simulink model "MotorGenerator1Basic_test_harness"  (R2022a)
settings: Solver=ode23t  StartTime=0.0  StopTime=t_end  RelTol=1e-3  AbsTol=1e-3
PreLoadFcn:
  | MotorGenerator1Basic_setup
undefined symbols (not defined in the file or in its folder): testharness
libraries: nesl_utility x3, fl_lib x1, sdl_lib x1
settings Model: Creator=isaacito  LastModifiedBy=isaacito
settings SolverCC: AutoScaleAbsTol=off  AlgebraicLoopSolver=TrustRegion
settings DebuggingCC: UnconnectedInputMsg=warning  UnconnectedOutputMsg=warning  UnconnectedLineMsg=warning  SymbolicDimsDataTypeCodeGenerationDiagnostic=none  SFMachineParentedDataDiag=warning
settings SFSimCC: CustomCodeUndefinedFunction=UseInterfaceOnly
settings RTWCC: DLArmComputeVersion=19.05
settings SimscapeCC: SimscapeLogType=all  SimscapeLogSimulationStatistics=on  SimscapeLogLimitData=off  SimscapeLogDataHistory=10000

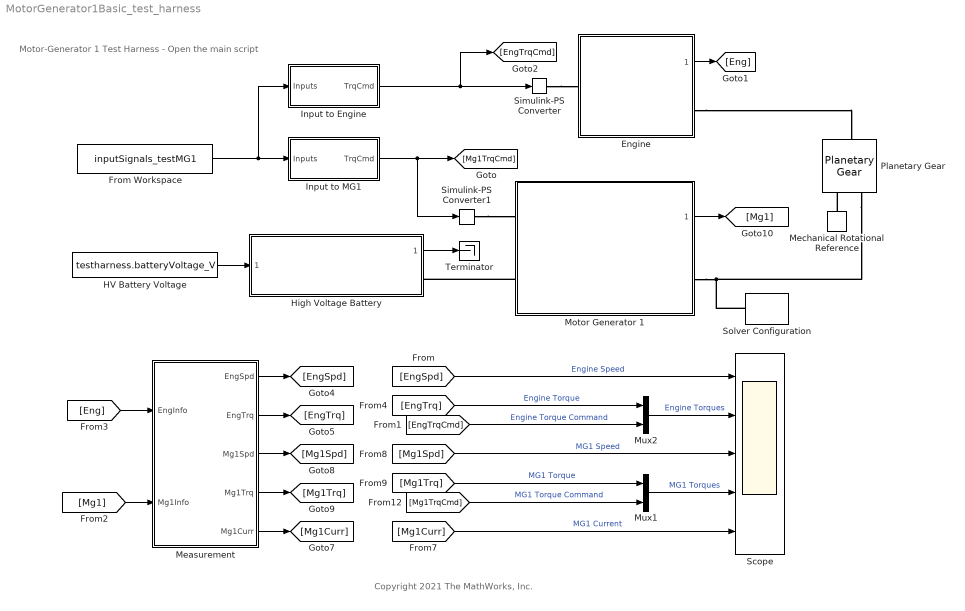
== system MotorGenerator1Basic_test_harness ==
  note: Copyright 2021 The MathWorks, Inc.
  note: Motor-Generator 1 Test Harness
      | - Open the main script
  Engine : Subsystem  ReferencedSubsystem=EngineBasic_refsub
      settings: PortSchema="{\"entries\":[{\"content\":{\"sides\":[{\"content\":{\"connectorIds\":[\"RConn1\"]},\"type\":\"ConnectorPlacement.EquallySpacedRectSide\",\"uuid\":\"5f0e7c9a-363d-4994-a013-d94ca7bd087a\"},{\"content\":{\"connectorIds\":[\"Out1\",\"LConn1\"],\"side\":\"RIGHT\"},\"type\":\"ConnectorPlacement.EquallySpacedRectSide\",\"uuid\":\"ebc3b24e-2640-42e1-8db7-715085fcccfd\"},{\"content\":{\"connectorIds\":[],\"side\":\"TOP\"},\"type\":\"ConnectorPlacement.EquallySpacedRectSide\",\"uuid\":\"348bf4c7-11ba-4351-a8af-87d33bf26f7f\"},{\"content\":{\"connectorIds\":[],\"side\":\"HIDDEN\"},\"type\":\"ConnectorPlacement.EquallySpacedRectSide\",\"uuid\":\"1cb82837-ca80-45c4-bec7-ac28580eadb7\"}]},\"type\":\"ConnectorPlacement.EquallySpacedConnector\",\"uuid\":\"6e937982-b0a5-454c-84b0-bd79245ef5fe\"}],\"packageUris\":[\"http://schema.mathworks.com/mf0/Connector/R2020b\"],\"version\":\"1.0\"}"
  From Workspace : FromWorkspace  VariableName=inputSignals_testMG1  OutDataTypeStr=Bus: inputBus_testMG1  Interpolate=off  OutputAfterFinalValue=Holding final value
      settings: AttributesFormatString=%<OutDataTypeStr>
  HV Battery Voltage : Constant  Value=testharness.batteryVoltage_V
  High Voltage Battery : Subsystem  ReferencedSubsystem=BatteryForTest_refsub
  Input to Engine : Subsystem
  Input to MG1 : Subsystem
  Measurement : Subsystem
  Mechanical Rotational Reference : fl_lib/Mechanical/Rotational Elements/Mechanical Rotational Reference
      settings: SourceProductBaseCode=PW,SS,VE
  Motor Generator 1 : Subsystem  ReferencedSubsystem=MotorGenerator1Basic_refsub
      settings: PortSchema="{\"entries\":[{\"content\":{\"sides\":[{\"content\":{\"connectorIds\":[\"LConn2\",\"LConn1\"]},\"type\":\"ConnectorPlacement.EquallySpacedRectSide\",\"uuid\":\"776eba5b-fa0b-476e-bc25-638ffdaad34f\"},{\"content\":{\"connectorIds\":[\"Out1\",\"RConn1\"],\"side\":\"RIGHT\"},\"type\":\"ConnectorPlacement.EquallySpacedRectSide\",\"uuid\":\"4f3a20f1-a757-4d58-af45-1ca561c570ae\"},{\"content\":{\"connectorIds\":[],\"side\":\"TOP\"},\"type\":\"ConnectorPlacement.EquallySpacedRectSide\",\"uuid\":\"92ea57c0-7c62-4e58-98f6-e0ae25305e81\"},{\"content\":{\"connectorIds\":[],\"side\":\"HIDDEN\"},\"type\":\"ConnectorPlacement.EquallySpacedRectSide\",\"uuid\":\"c19be4f7-c21d-4f93-a091-e01cfe3eb863\"}]},\"type\":\"ConnectorPlacement.EquallySpacedConnector\",\"uuid\":\"27ec3241-2d74-4878-8a97-99674a624e01\"}],\"packageUris\":[\"http://schema.mathworks.com/mf0/Connector/R2020b\"],\"version\":\"1.0\"}"
  Mux1 : Mux  Inputs=2
  Mux2 : Mux  Inputs=2
  Planetary Gear : sdl_lib/Gears/Planetary Gear  rs_ratio=powerSplit.planetary_ringToSunGearRatio  friction_model=sdl.enum.gear_friction.constant  efficiency=powerSplit.planetary_efficiencies  temperature_TLU=[280, 300, 320] K  efficiency_sp_TLU=[.95, .9, .85]  efficiency_rp_TLU=[.95, .9, .85]  pwr_thr=smoothing.planetary_meshing_loss_thresholds_W W  mu_visc=powerSplit.planetary_frictions_Nm_per_rpm m*N/rpm  model_inertia=simscape.enum.onoff.on  planet_inertia=powerSplit.planetary_planetGearInertia_kg_m2 kg*m^2  thermal_mass=50 J/K  T_init=300 K
      settings: SourceProductBaseCode=LD
  Scope : Scope  NumInputPorts=5
  Simulink-PS Converter : nesl_utility/Simulink-PS Converter  PhysicalDomain=network_engine_domain  SubClassName=ps_input  LeftPortType=input  RightPortType=output  PseudoPeriodic=off  Frequencies=[]  NoiseDistribution=none  NoiseParameters=[]  Unit=N*m  AffineConversion=off  FilteringAndDerivatives=provide  SimscapeFilterOrder=1  InputFilterTimeConstant=0.001  UdotUserProvided=0
      settings: SourceProductName=Utilities
  Simulink-PS Converter1 : nesl_utility/Simulink-PS Converter  PhysicalDomain=network_engine_domain  SubClassName=ps_input  LeftPortType=input  RightPortType=output  PseudoPeriodic=off  Frequencies=[]  NoiseDistribution=none  NoiseParameters=[]  Unit=N*m  AffineConversion=off  FilteringAndDerivatives=provide  SimscapeFilterOrder=1  InputFilterTimeConstant=0.001  UdotUserProvided=0
      settings: SourceProductName=Utilities
  Solver Configuration : nesl_utility/Solver Configuration  PhysicalDomain=network_engine_domain  SubClassName=solver  LeftPortType=input  RightPortType=generic  Tones=[]  Harmonics=[]  SimulateNoise=off  Profile=off  UseLocalSampling=off  EnableSwitchedLinearOptims=on  FrequencyDomain=off  UseCCode=off  RelTol=0.001  AbsTol=1e-06  MinStep=1e-09  ToWorkspace=off  RevertToSquareIcSolve=off  NumHomotopyIterations=100  PhasorMode=off  PhasorModeNumHarmonics=1  IndexReductionMethod=DerivativeReplacement  DoDC=off  ResidualTolerance=1e-09  UseLocalSolver=off  LocalSolverChoice=NE_BACKWARD_EULER_ADVANCER  LocalSolverSampleTime=0.001  DoFixedCost=off  MaxNonlinIter=3  MaxModeIter=2  ComputeImpulses=off  ImpulseIterations=2  LinearAlgebra=auto  LinearAlgebraNumThread=0  EquationFormulation=NE_TIME_EF  DelaysMemoryBudget=1024  AutomaticFiltering=on  FilteringTimeConstant=0.001  PartitionStorageMethod=AS_NEEDED  PartitionMemoryBudget=1024  PartitionMethod=ROBUST
      settings: SourceProductName=Utilities
  Terminator : Terminator
  wires:
  HV Battery Voltage/1 -> High Voltage Battery/1
  [Eng] -> Measurement/1(EngInfo)
  [Mg1] -> Measurement/2(Mg1Info)
  Measurement/1(EngSpd) -> [EngSpd]
  Measurement/2(EngTrq) -> [EngTrq]
  Measurement/5(Mg1Curr) -> [Mg1Curr]
  Measurement/3(Mg1Spd) -> [Mg1Spd]
  Measurement/4(Mg1Trq) -> [Mg1Trq]
  [Mg1TrqCmd] -> Mux1/2  "MG1 Torque Command"
  [Mg1Trq] -> Mux1/1  "MG1 Torque"
  Input to Engine/1(TrqCmd) -> [EngTrqCmd], Simulink-PS Converter/1
  Engine/1 -> [Eng]
  [EngTrq] -> Mux2/1  "Engine Torque"
  [EngTrqCmd] -> Mux2/2  "Engine Torque Command"
  [EngSpd] -> Scope/1  "Engine Speed"
  Mux2/1 -> Scope/2  "Engine Torques"
  Mux1/1 -> Scope/4  "MG1 Torques"
  [Mg1Curr] -> Scope/5  "MG1 Current"
  From Workspace/1 -> Input to Engine/1(Inputs), Input to MG1/1(Inputs)
  Input to MG1/1(TrqCmd) -> [Mg1TrqCmd], Simulink-PS Converter1/1
  [Mg1Spd] -> Scope/3  "MG1 Speed"
  Motor Generator 1/1 -> [Mg1]
  High Voltage Battery/1 -> Terminator/1
  connections:
  Simulink-PS Converter/RConn1 -- Engine/RConn1
  Mechanical Rotational Reference/LConn1 -- Planetary Gear/RConn1
  Engine/LConn1 -- Planetary Gear/LConn1
  Planetary Gear/RConn2 -- Motor Generator 1/RConn1 -- Solver Configuration/RConn1
  Motor Generator 1/LConn1 -- High Voltage Battery/RConn1
  Simulink-PS Converter1/RConn1 -- Motor Generator 1/LConn2

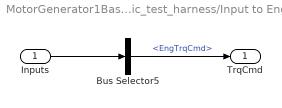
== system MotorGenerator1Basic_test_harness/Input to Engine ==
  Inputs : Inport
  Bus Selector5 : BusSelector  OutputSignals=EngTrqCmd
  TrqCmd : Outport
  wires:
  Bus Selector5/1 -> TrqCmd/1  "<EngTrqCmd>"
  Inputs/1 -> Bus Selector5/1

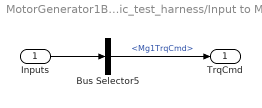
== system MotorGenerator1Basic_test_harness/Input to MG1 ==
  Inputs : Inport
  Bus Selector5 : BusSelector  OutputSignals=Mg1TrqCmd
  TrqCmd : Outport
  wires:
  Bus Selector5/1 -> TrqCmd/1  "<Mg1TrqCmd>"
  Inputs/1 -> Bus Selector5/1

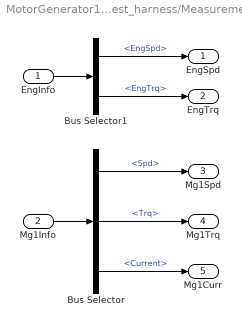
== system MotorGenerator1Basic_test_harness/Measurement ==
  EngInfo : Inport
  Mg1Info : Inport  Port=2
  Bus Selector : BusSelector  OutputSignals=Spd,Trq,Current
  Bus Selector1 : BusSelector  OutputSignals=EngSpd,EngTrq
  EngSpd : Outport
  EngTrq : Outport  Port=2
  Mg1Spd : Outport  Port=3
  Mg1Trq : Outport  Port=4
  Mg1Curr : Outport  Port=5
  wires:
  EngInfo/1 -> Bus Selector1/1
  Bus Selector1/1 -> EngSpd/1  "<EngSpd>"
  Bus Selector1/2 -> EngTrq/1  "<EngTrq>"
  Mg1Info/1 -> Bus Selector/1
  Bus Selector/1 -> Mg1Spd/1  "<Spd>"
  Bus Selector/2 -> Mg1Trq/1  "<Trq>"
  Bus Selector/3 -> Mg1Curr/1  "<Current>"
